simulink model "simulink_model"  (R2021b)
settings: Solver=FixedStepAuto  StartTime=0.0  StopTime=inf  RelTol=1e-3  EnableMultiTasking=on
libraries: arduinolib x4, cstblocks x2
settings Model: ExtModeTrigDuration=2  Creator=Admin  LastModifiedBy=Admin
settings OptimizationCC: EnhancedBackFolding=on  PassReuseOutputArgsAs=Individual arguments  ZeroExternalMemoryAtStartup=off  ZeroInternalMemoryAtStartup=off  MaxStackSize=64  OptimizeBlockOrder=speed  DifferentSizesBufferReuse=on  OptimizationCustomize=off  EfficientTunableParamExpr=on
settings DebuggingCC: ParameterTunabilityLossMsg=error
settings HardwareCC: ProdBitPerInt=16  ProdBitPerPointer=16  ProdBitPerSizeT=16  ProdBitPerPtrDiffT=16  ProdLargestAtomicFloat=None  ProdWordSize=8  ProdHWDeviceType=Atmel->AVR  UseEmbeddedCoderFeatures=off  UseSimulinkCoderFeatures=off
settings SFSimCC: MATLABDynamicMemAlloc=off
settings RTWCC: Description=Embedded Coder  SystemTargetFile=ert.tlc  HardwareBoard=Arduino Mega 2560  TemplateMakefile=ert_default_tmf  Toolchain=Arduino AVR  BuildConfiguration=Faster Runs
settings CodeAppCC: ForceParamTrailComments=on  IgnoreCustomStorageClasses=off  OperatorAnnotations=on  SimulinkDataObjDesc=on  SFDataObjDesc=on  InsertBlockDesc=on
settings ERTTargetCC: SupportContinuousTime=on  SupportNonInlinedSFcns=on  SupportVariableSizeSignals=on  ExtModeTransport=3  ExtModeStaticAlloc=on  ExtModeStaticAllocSize=2048  ExtModeMexFile=ext_xcp  ExtModeIntrfLevel=Level2 - Open

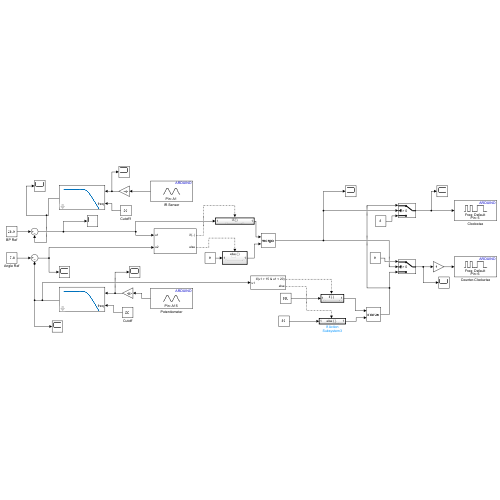
[thumbnail: Simulink's stored preview of the top-level diagram]
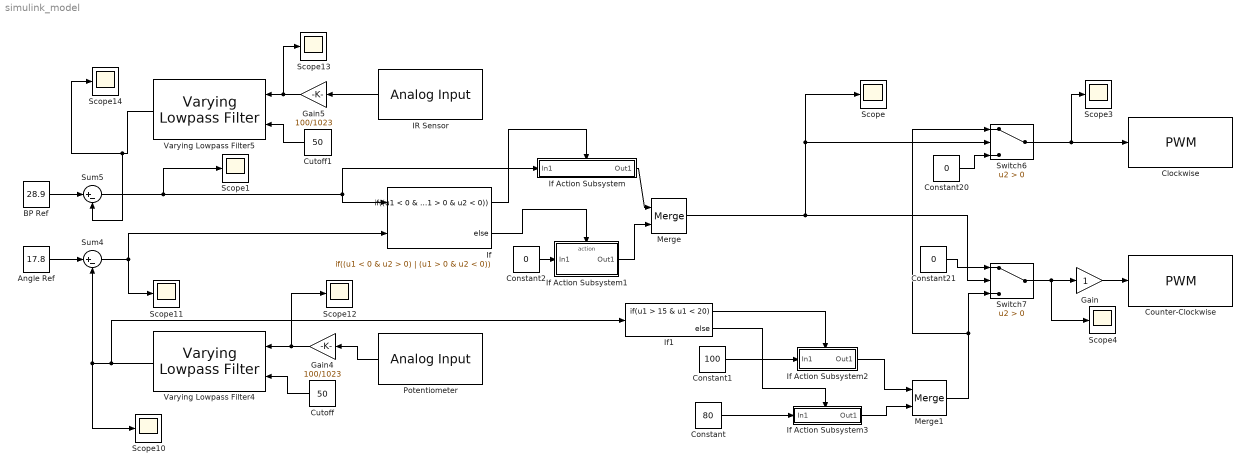
== system simulink_model ==
  Angle Ref : Constant  Value=17.8  SampleTime=0.001
  BP Ref : Constant  Value=28.9  SampleTime=0.001
  Clockwise : arduinolib/PWM  pinNumber=5  frequencyType=Default  desiredFrequency=490.2  achievableFrequency=490.2
  Constant : Constant  Value=80
  Constant1 : Constant  Value=100
  Constant2 : Constant  Value=0
  Constant20 : Constant  Value=0  SampleTime=0.001
  Constant21 : Constant  Value=0  SampleTime=0.001
  Counter-Clockwise : arduinolib/PWM  pinNumber=6  frequencyType=Default  desiredFrequency=490.2  achievableFrequency=490.2
  Cutoff : Constant  Value=50  SampleTime=0.001
  Cutoff1 : Constant  Value=50  SampleTime=0.001
  Gain : Gain
  Gain4 : Gain  Gain=100/1023
  Gain5 : Gain  Gain=100/1023
  IR Sensor : arduinolib/Analog Input  pinNumber=1  ReadResultsOnly=off  ConversionTriggerSource=Software  ExternalTriggerType=uint32( 0 )  OutputDataType=uint16  EnableConversionCompleteNotify=off  EnableOuputStatus=off  SampleTime=0.001  blockPlatform=arduino
  If : If  NumInputs=2  IfExpression=(u1 < 0 & u2 > 0) | (u1 > 0 & u2 < 0)
  If Action Subsystem : Subsystem  TreatAsAtomicUnit=on
  If Action Subsystem1 : Subsystem  TreatAsAtomicUnit=on
  If Action Subsystem2 : Subsystem  TreatAsAtomicUnit=on
  If Action Subsystem3 : Subsystem  TreatAsAtomicUnit=on
  If1 : If  IfExpression=u1 > 15 & u1 < 20
  Merge : Merge
  Merge1 : Merge
  Potentiometer : arduinolib/Analog Input  pinNumber=15  ReadResultsOnly=off  ConversionTriggerSource=Software  ExternalTriggerType=uint32( 0 )  OutputDataType=uint16  EnableConversionCompleteNotify=off  EnableOuputStatus=off  SampleTime=0.001  blockPlatform=arduino
  Scope{,1,3..4,10..14} (9 alike) : Scope
  Sum4 : Sum  Inputs=|+-
  Sum5 : Sum  Inputs=|+-
  Switch6 : Switch  Criteria=u2 > Threshold
  Switch7 : Switch  Criteria=u2 > Threshold
  Varying Lowpass Filter4 : cstblocks/Linear Parameter Varying/Varying Lowpass Filter  N=1
  Varying Lowpass Filter5 : cstblocks/Linear Parameter Varying/Varying Lowpass Filter  N=1
  wires:
  Sum5/1 -> If/1, If Action Subsystem/1(In1), Scope1/1
  Cutoff1/1 -> Varying Lowpass Filter5/2
  IR Sensor/1 -> Gain5/1
  Gain5/1 -> Scope13/1, Varying Lowpass Filter5/1
  Gain4/1 -> Scope12/1, Varying Lowpass Filter4/1
  Sum4/1 -> Scope11/1, If/2
  Constant20/1 -> Switch6/3
  Varying Lowpass Filter5/1 -> Scope14/1, Sum5/2
  Cutoff/1 -> Varying Lowpass Filter4/2
  BP Ref/1 -> Sum5/1
  Varying Lowpass Filter4/1 -> If1/1, Scope10/1, Sum4/2
  Angle Ref/1 -> Sum4/1
  Switch6/1 -> Scope3/1, Clockwise/1
  Switch7/1 -> Gain/1, Scope4/1
  Constant21/1 -> Switch7/1
  Potentiometer/1 -> Gain4/1
  If Action Subsystem/1(Out1) -> Merge/1
  If/1 -> If Action Subsystem/Action
  If/2 -> If Action Subsystem1/Action
  Constant2/1 -> If Action Subsystem1/1(In1)
  If Action Subsystem1/1(Out1) -> Merge/2
  Gain/1 -> Counter-Clockwise/1
  Merge/1 -> Switch7/2, Scope/1, Switch6/2
  If1/1 -> If Action Subsystem2/Action
  Constant1/1 -> If Action Subsystem2/1(In1)
  If1/2 -> If Action Subsystem3/Action
  Constant/1 -> If Action Subsystem3/1(In1)
  If Action Subsystem2/1(Out1) -> Merge1/1
  If Action Subsystem3/1(Out1) -> Merge1/2
  Merge1/1 -> Switch6/1, Switch7/3

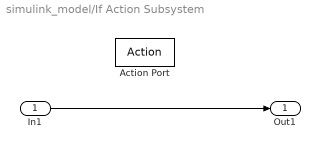
== system simulink_model/If Action Subsystem ==
  In1 : Inport
  Action Port : ActionPort  ActionPortLabel=if((u1 < 0 & u2 > 0) | (u1 > 0 & u2 < 0))
  Out1 : Outport
  wires:
  In1/1 -> Out1/1

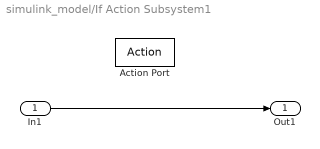
== system simulink_model/If Action Subsystem1 ==
  In1 : Inport
  Action Port : ActionPort  ActionPortLabel=else
  Out1 : Outport
  wires:
  In1/1 -> Out1/1

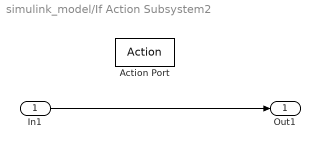
== system simulink_model/If Action Subsystem2 ==
  In1 : Inport
  Action Port : ActionPort  ActionPortLabel=if(u1 > 15 & u1 < 20)
  Out1 : Outport
  wires:
  In1/1 -> Out1/1

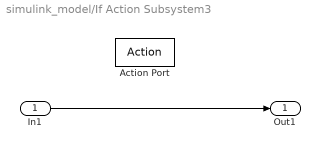
== system simulink_model/If Action Subsystem3 ==
  In1 : Inport
  Action Port : ActionPort  ActionPortLabel=else
  Out1 : Outport
  wires:
  In1/1 -> Out1/1
